simulink model "gm_hdl_model_fixed"  (R2024a)
settings: Solver=FixedStepDiscrete  StartTime=0.0  StopTime=SIM_TIME  RelTol=1e-3
undefined symbols (not defined in the file or in its folder): a, b, BUFFER_LEN, c, SAMPLING_FREQ, signal_1
libraries: hdlsllib x39, dspsigops x15, simulink_extras x4, simulink x2, dspsrcs4 x1, dsphdlxfrm2 x1
(part 3 of 3)

== system gm_hdl_model_fixed/Subsystem1/Subsystem Reference/Real Divide HDL Optimized/ForEach - Real Divide_instance1/Normalize numerator/positiveRealNormalizer/embreciprocals_c3_positiveRealNormalizer_controlled ==
  in0 : Inport  OutDataTypeStr=fixdt(1, 17, 14)  SampleTime=1e-08
  in1 : Inport  Port=2  OutDataTypeStr=boolean  SampleTime=1e-08
  stateControl : EnablePort  OutDataTypeStr=boolean
  embreciprocals_c3_positiveRealNormalizer : MATLAB Function  TreatAsAtomicUnit=on
      settings: LibrarySourceBlock=embreciprocals/Real Normalizer HDL Optimized/positiveRealNormalizer
  out0 : Outport  OutDataTypeStr=fixdt(1, 17, 15)  SampleTime=1e-08  InitialOutput=0
  out1 : Outport  Port=2  OutDataTypeStr=int32  SampleTime=1e-08  InitialOutput=0
  out2 : Outport  Port=3  OutDataTypeStr=boolean  SampleTime=1e-08  InitialOutput=0
  out3 : Outport  Port=4  OutDataTypeStr=boolean  SampleTime=1e-08  InitialOutput=0
  wires:
  embreciprocals_c3_positiveRealNormalizer/1(x) -> out0/1
  embreciprocals_c3_positiveRealNormalizer/2(e) -> out1/1
  embreciprocals_c3_positiveRealNormalizer/3(isNegative) -> out2/1
  embreciprocals_c3_positiveRealNormalizer/4(validOut) -> out3/1
  in0/1 -> embreciprocals_c3_positiveRealNormalizer/1(u)
  in1/1 -> embreciprocals_c3_positiveRealNormalizer/2(validIn)

== matlab function gm_hdl_model_fixed/Subsystem1/Subsystem Reference/Real Divide HDL Optimized/ForEach - Real Divide_instance1/Upcast Wordlength/slutils_c2_Upcast_Wordlength ==
  data: x input; u output; y input; v output
function [u, v] = upcastWordlength(x, y)

% Copyright 2019 The MathWorks, Inc.

%#codegen

[u, v] = fixed.internal.type.upcastWordlength(x,y);

end

== matlab function gm_hdl_model_fixed/Subsystem1/Subsystem Reference/Real Divide HDL Optimized/Reshape to original size/embreciprocals_c11_Reshape_to_original_size ==
  data: y input; u input; z output
function z = reshape_to_original_size(y,u)
    z = reshape(y,size(u));
end

== matlab function gm_hdl_model_fixed/Subsystem1/myRMS/CORDIC Square Root HDL Optimized/Synchronous Subsystem/cordicSquareRootHDL/embmathops_c2_s84XJG1CWMolALoedlonStG_cordicSquareRootHDL_controlled/embmathops_c2_s84XJG1CWMolALoedlonStG_cordicSquareRootHDL ==
  settings: fimath=hdlfimath
  data: u input; dataOut output; validIn input; restart input; eOut output; isZero output; validOut output; maximumShiftValue parameter; nIterPerReg parameter; autoMaximumShiftVal parameter
function [dataOut,eOut,isZero,validOut] = cordicSquareRootHDL(u,validIn,restart,maximumShiftValue, nIterPerReg, autoMaximumShiftVal)
    % [dataOut,eOut,validOut] = cordicSquareRootHDL(u,validIn,restart,maximumShiftValue,nIterPerReg)
    % This function computes the normalized square root of input data u
    % based on CORDIC hyperbolic vectoring mode. eOut is the bit shift
    % value to be used during denormalization.
    %
    % This function first performs normalization of input u and then
    % computes square root of normalized u using CORDIC hyperbolic
    % vectoring mode.

    %   Copyright 2023 The MathWorks, Inc.

    %#codegen
    
    fixed.internal.reciprocal.validateNormalizerInputs(u, validIn);

    %% Constants
    if autoMaximumShiftVal
        N = coder.const(fixed.cordic.maximumShiftValue(u));
    else
        N = coder.const(maximumShiftValue);
    end

    Kn = coder.const(fixed.cordic.hyperbolic.inverseScaleFactor(N));
    INITOFFSET = coder.const(0.25);
    shiftSeq = coder.const(fixed.cordic.hyperbolic.shiftSequence(N));
    nCORDICIterations = coder.const(length(shiftSeq));

    %% Run CORDIC square root workflow
    uPos = fixed.cordic.linear.makeRealScalarPositiveUnsigned(u);
    if isfi(u)&&isscaledtype(u)
        coder.internal.assert(u.WordLength>N,'fixed:emblib:CORDICMaxShiftValMustBeSmallerThanWordlength');
        [dataOut, eOut, isZero, validOut] = sqrtIterFixed(uPos, validIn, restart,nIterPerReg,Kn,INITOFFSET,shiftSeq,nCORDICIterations);
    else
        [dataOut, eOut] = fixed.emblib.cordicsqrt.cordicSqrtFloat(uPos, Kn, INITOFFSET, shiftSeq, nCORDICIterations);
        validOut = validIn;
        isZero = u==0;
    end
end

function [dataOut, eOut, isZero, validOut] = sqrtIterFixed(u, validIn, restart, nIterPerReg, Kn, INITOFFSET, shiftSeq, nCORDICIterations)
        uInt = stripscaling(u);
        
        wordLength = coder.const(uInt.WordLength);
        normalizerType = numerictype(1,32,0);

        % CORDIC datatype and corresponding fimath
        CORDICprototype = fi([],1,wordLength,wordLength-2,'DataType',uInt.DataType);
        Fxy = fixed.fimathLike(CORDICprototype);
        
        % Allocate registers
        [numOfNormSteps,nNormReg,normInd,nTrailingNormSteps,trailingNormIdx,nLeadingCORDICSteps,nCORDICReg,CORDICShiftInd,nTotReg]...
            = fixed.emblib.cordicsqrt.allocateReg(wordLength,nCORDICIterations,nIterPerReg);
        
        %% Registers
        persistent xRegNorm xRegCORDIC yReg eRegNorm eRegCORDIC validReg dataOutReg eOutReg isZeroReg
        if isempty(xRegNorm)
            xRegNorm = zeros(nNormReg,1,'like',uInt);
            xRegCORDIC = setfimath(zeros(nCORDICReg,1,'like',CORDICprototype),Fxy);
            yReg = setfimath(zeros(nCORDICReg,1,'like',CORDICprototype),Fxy);
            eRegNorm = fi(zeros(nNormReg,1),0,numOfNormSteps,0);
            eRegCORDIC = fi(zeros(nCORDICReg,1),normalizerType);
            validReg = false(nTotReg+1,1);
            dataOutReg = setfimath(cast(0,'like',CORDICprototype),Fxy);
            eOutReg = fi(0,normalizerType);
            isZeroReg = false(nTotReg+1,1);
        end
        
        %% Assign outputs
        dataOut = dataOutReg;
        eOut = eOutReg;
        validOut = validReg(end);
        isZero = isZeroReg(end);
        
        %% Update registers
        [xRegNorm, xRegCORDIC, yReg, eRegNorm, eRegCORDIC, validReg, dataOutReg, eOutReg, isZeroReg]...
        = fixed.emblib.cordicsqrt.cordicSqrtFiScaledtypeUpdateReg(u, uInt, validIn, restart,... % Inputs
        xRegNorm, xRegCORDIC, yReg, eRegNorm, eRegCORDIC, validReg, dataOutReg, eOutReg, isZeroReg,... %Registers
        Kn, INITOFFSET, shiftSeq, nIterPerReg,... % Constants for algorithms
        nTotReg, nNormReg, CORDICShiftInd, normInd, nTrailingNormSteps, trailingNormIdx, nLeadingCORDICSteps); % Constants for partition algorithms
end

== matlab function gm_hdl_model_fixed/Subsystem1/Subsystem Reference/Real Divide HDL Optimized/ForEach - Real Divide_instance1/MATLAB Function/embreciprocals_c13_MATLAB_Function ==
  settings: fimath=hdlfimath
  data: num input; num_out output; t_num input; t_num_out output
function [num_out, t_num_out] = fcn(num, t_num)

num_out = bitsra(num,1);
t_num_out = t_num - 1;

end

== matlab function gm_hdl_model_fixed/Subsystem1/myRMS/CORDIC Square Root HDL Optimized/Cast to Union of Types/slutils_c1_sjX4rJHbVvOr6YSpugZXv9B_Cast_to_Union_of_Types ==
  settings: fimath=hdlfimath
  data: Xref input; Cout output; Cin input
function Cout = castToUnionType(Xref,Cin)
    %castToUnionType Cast second input to union of the two types
    if (isfloat(Xref) && isfloat(Cin)) || (isFixed(Xref) && isFixed(Cin))
        T = fixed.internal.type.unionPrototype(Cin,Xref,...
        'RoundingMethod','Floor',...
        'OverflowAction','Wrap');
        Cout = cast(Cin,'like',T);
    else
        coder.internal.assert(false,'fixed:emblib:InputOutputMustBeAllFixedOrFloat');
    end
end

function t = isFixed(x)
    t = (isfi(x) || isa(x,'embedded.numerictype')) && isscalingbinarypoint(x) ...
        || isinteger(x);
end

== matlab function gm_hdl_model_fixed/Subsystem1/myRMS/CORDIC Square Root HDL Optimized/Bit Shift Arithmetic/embmathops_c6_st99WwhDyWfnOmuPiiKPkxE_Bit_Shift_Arithmetic ==
  settings: fimath=hdlfimath
  data: u input; y output; e input; isZero input
function y = bitShiftArithmetic(u,e,isZero)
%#codegen
if isZero
    y = cast(0,'like',u);
else
    if e<0
        y = bitsll(u,-e);
    else
        y = bitsra(u,e);
    end
end

== matlab function gm_hdl_model_fixed/Subsystem1/Subsystem Reference/Absolute of Complex/CORDIC Square Root HDL Optimized1/Cast to Union of Types/slutils_c1_sJq36p6JfwxqYYDPRgb8M6G_Cast_to_Union_of_Types ==
  settings: fimath=hdlfimath
  data: Xref input; Cout output; Cin input
function Cout = castToUnionType(Xref,Cin)
    %castToUnionType Cast second input to union of the two types
    if (isfloat(Xref) && isfloat(Cin)) || (isFixed(Xref) && isFixed(Cin))
        T = fixed.internal.type.unionPrototype(Cin,Xref,...
        'RoundingMethod','Floor',...
        'OverflowAction','Wrap');
        Cout = cast(Cin,'like',T);
    else
        coder.internal.assert(false,'fixed:emblib:InputOutputMustBeAllFixedOrFloat');
    end
end

function t = isFixed(x)
    t = (isfi(x) || isa(x,'embedded.numerictype')) && isscalingbinarypoint(x) ...
        || isinteger(x);
end

== matlab function gm_hdl_model_fixed/Subsystem1/Subsystem Reference/Real Divide HDL Optimized/y = u(1)/embreciprocals_c16_y___u_1_ ==
  data: u input; y output
function y = select_one(u)
    y = u(1);
end

== matlab function gm_hdl_model_fixed/Subsystem1/Subsystem Reference/Real Divide HDL Optimized/Verify divide sizes/embreciprocals_c19_Verify_divide_sizes ==
  data: denominator input; den output; numerator input; num output
function [den,num] = verify_size(denominator,numerator)
   % Verify that the dimensions of the input arrays match, and then reshape
   % them.
   coder.internal.assert(numel(denominator)==numel(numerator),...
       'fixed:emblib:DivideDimensionsShouldMatch',...
       'Real Divide HDL Optimized');
   num = reshape(numerator,1,numel(numerator));
   den = reshape(denominator,1,numel(denominator));
end

== matlab function gm_hdl_model_fixed/Subsystem1/Subsystem Reference/Real Divide HDL Optimized/ForEach - Real Divide_instance1/Divide real numerator by denominator/normalizedCORDICDivide/embreciprocals_c21_normalizedCORDICDivide_controlled/embreciprocals_c21_normalizedCORDICDivide ==
  settings: fimath=hdlfimath
  data: num input; den input; tNum input; tDen input; isNumNegative input; isDenNegative input; y output; t output; isDenZeroOut output; validIn input; validOut output
function [y, t, isDenZeroOut, validOut] = normalizedCORDICDivide(num, den, tNum, tDen, isNumNegative, isDenNegative, validIn)
    %   Copyright 2020 The MathWorks, Inc.
    %#codegen
    fixed.internal.reciprocal.validateReciprocalInputs(num, validIn);
    if isfi(num) && isscaledtype(num)
        isDenZero = den==0;
        isNumZero = num==0;
        % CORDIC divide for fixed-point and scaled-double types
        [y,t,isNegative,isNumZeroOut, isDenZeroOut,validOut] = fixedpointDivide(den,num,tDen-tNum,isNumNegative ~= isDenNegative, isNumZero, isDenZero,validIn);
    else
        % y = num/den for builtin types.
        y = num./den;
        t = tDen - tNum;
        isNegative = isNumNegative ~= isDenNegative;
        validOut = validIn;
        isDenZeroOut = false;
        isNumZeroOut = false;
    end
    if isNumZeroOut
        % Negate with saturate so the most negative value doesn't overflow.
        F = fimath('OverflowAction', 'Saturate');
        y(:) = setfimath(0,F);
    else
        if isNegative
            % Negate with saturate so the most negative value doesn't overflow.
            F = fimath('OverflowAction', 'Saturate');
            y(:) = -setfimath(y,F);
        end
    end
end

function [division, t, isNegativeOut, isNumZeroOut, isDenZeroOut, validOut] = fixedpointDivide(x,y,t_in,isNegative,isNumZero,isDenZero,validIn)
    T = fixed.cordic.linear.positiveReciprocalTypes(x);
    maximumShiftValue = coder.const(fixed.cordic.maximumShiftValue(T.data));
    % Register variables for the CORDIC Divide Kernel
    persistent xReg yReg zReg validReg tReg isNegativeReg isNumZeroReg isDenZeroReg
    if isempty(xReg)
        xReg = zeros(maximumShiftValue+2,1,'like',T.data);
        yReg = zeros(maximumShiftValue+2,1,'like',T.data);
        zReg = zeros(maximumShiftValue+2,1,'like',T.data);
        validReg = zeros(maximumShiftValue+2,1,'like',validIn);
        tReg = zeros(maximumShiftValue+2,1,'like',t_in);
        isNegativeReg = false(maximumShiftValue+2,1);
        isDenZeroReg = false(maximumShiftValue+2,1);
        isNumZeroReg = false(maximumShiftValue+2,1);
    end
    % CORDIC Divide Kernel
    [division,t,validOut,...
        xReg,yReg,zReg,validReg,tReg... % Persistent variables
        ] = fixed.internal.reciprocal.cordicDivideKernel(x,y,t_in,validIn,...
        xReg,yReg,zReg,validReg,tReg... % Persistent variables
        );
    
    % Assign outputs from states
    isNegativeOut = isNegativeReg(end);
    isNumZeroOut = isNumZeroReg(end);
    isDenZeroOut = isDenZeroReg(end);
    % Update isNegative states
    coder.unroll
    for k = maximumShiftValue+1:-1:1
        isNegativeReg(k+1) = isNegativeReg(k);
        isNumZeroReg(k+1) = isNumZeroReg(k);
        isDenZeroReg(k+1) = isDenZeroReg(k);
    end
    isNegativeReg(1) = isNegative;
    isNumZeroReg(1) = isNumZero;
    isDenZeroReg(1) = isDenZero;
end

== matlab function gm_hdl_model_fixed/Subsystem1/Subsystem Reference/Absolute of Complex/CORDIC Square Root HDL Optimized1/Synchronous Subsystem/cordicSquareRootHDL/embmathops_c2_srwrzER3uCGRdPfDbow0ID_cordicSquareRootHDL_controlled/embmathops_c2_srwrzER3uCGRdPfDbow0ID_cordicSquareRootHDL ==
  settings: fimath=hdlfimath
  data: u input; dataOut output; validIn input; restart input; eOut output; isZero output; validOut output; maximumShiftValue parameter; nIterPerReg parameter; autoMaximumShiftVal parameter
function [dataOut,eOut,isZero,validOut] = cordicSquareRootHDL(u,validIn,restart,maximumShiftValue, nIterPerReg, autoMaximumShiftVal)
    % [dataOut,eOut,validOut] = cordicSquareRootHDL(u,validIn,restart,maximumShiftValue,nIterPerReg)
    % This function computes the normalized square root of input data u
    % based on CORDIC hyperbolic vectoring mode. eOut is the bit shift
    % value to be used during denormalization.
    %
    % This function first performs normalization of input u and then
    % computes square root of normalized u using CORDIC hyperbolic
    % vectoring mode.

    %   Copyright 2023 The MathWorks, Inc.

    %#codegen
    
    fixed.internal.reciprocal.validateNormalizerInputs(u, validIn);

    %% Constants
    if autoMaximumShiftVal
        N = coder.const(fixed.cordic.maximumShiftValue(u));
    else
        N = coder.const(maximumShiftValue);
    end

    Kn = coder.const(fixed.cordic.hyperbolic.inverseScaleFactor(N));
    INITOFFSET = coder.const(0.25);
    shiftSeq = coder.const(fixed.cordic.hyperbolic.shiftSequence(N));
    nCORDICIterations = coder.const(length(shiftSeq));

    %% Run CORDIC square root workflow
    uPos = fixed.cordic.linear.makeRealScalarPositiveUnsigned(u);
    if isfi(u)&&isscaledtype(u)
        coder.internal.assert(u.WordLength>N,'fixed:emblib:CORDICMaxShiftValMustBeSmallerThanWordlength');
        [dataOut, eOut, isZero, validOut] = sqrtIterFixed(uPos, validIn, restart,nIterPerReg,Kn,INITOFFSET,shiftSeq,nCORDICIterations);
    else
        [dataOut, eOut] = fixed.emblib.cordicsqrt.cordicSqrtFloat(uPos, Kn, INITOFFSET, shiftSeq, nCORDICIterations);
        validOut = validIn;
        isZero = u==0;
    end
end

function [dataOut, eOut, isZero, validOut] = sqrtIterFixed(u, validIn, restart, nIterPerReg, Kn, INITOFFSET, shiftSeq, nCORDICIterations)
        uInt = stripscaling(u);
        
        wordLength = coder.const(uInt.WordLength);
        normalizerType = numerictype(1,32,0);

        % CORDIC datatype and corresponding fimath
        CORDICprototype = fi([],1,wordLength,wordLength-2,'DataType',uInt.DataType);
        Fxy = fixed.fimathLike(CORDICprototype);
        
        % Allocate registers
        [numOfNormSteps,nNormReg,normInd,nTrailingNormSteps,trailingNormIdx,nLeadingCORDICSteps,nCORDICReg,CORDICShiftInd,nTotReg]...
            = fixed.emblib.cordicsqrt.allocateReg(wordLength,nCORDICIterations,nIterPerReg);
        
        %% Registers
        persistent xRegNorm xRegCORDIC yReg eRegNorm eRegCORDIC validReg dataOutReg eOutReg isZeroReg
        if isempty(xRegNorm)
            xRegNorm = zeros(nNormReg,1,'like',uInt);
            xRegCORDIC = setfimath(zeros(nCORDICReg,1,'like',CORDICprototype),Fxy);
            yReg = setfimath(zeros(nCORDICReg,1,'like',CORDICprototype),Fxy);
            eRegNorm = fi(zeros(nNormReg,1),0,numOfNormSteps,0);
            eRegCORDIC = fi(zeros(nCORDICReg,1),normalizerType);
            validReg = false(nTotReg+1,1);
            dataOutReg = setfimath(cast(0,'like',CORDICprototype),Fxy);
            eOutReg = fi(0,normalizerType);
            isZeroReg = false(nTotReg+1,1);
        end
        
        %% Assign outputs
        dataOut = dataOutReg;
        eOut = eOutReg;
        validOut = validReg(end);
        isZero = isZeroReg(end);
        
        %% Update registers
        [xRegNorm, xRegCORDIC, yReg, eRegNorm, eRegCORDIC, validReg, dataOutReg, eOutReg, isZeroReg]...
        = fixed.emblib.cordicsqrt.cordicSqrtFiScaledtypeUpdateReg(u, uInt, validIn, restart,... % Inputs
        xRegNorm, xRegCORDIC, yReg, eRegNorm, eRegCORDIC, validReg, dataOutReg, eOutReg, isZeroReg,... %Registers
        Kn, INITOFFSET, shiftSeq, nIterPerReg,... % Constants for algorithms
        nTotReg, nNormReg, CORDICShiftInd, normInd, nTrailingNormSteps, trailingNormIdx, nLeadingCORDICSteps); % Constants for partition algorithms
end

== matlab function gm_hdl_model_fixed/Subsystem1/Subsystem Reference/CORDIC Square Root HDL Optimized/Synchronous Subsystem/cordicSquareRootHDL/embmathops_c2_skVmLPFzLIK224pVNfQB1qF_cordicSquareRootHDL_controlled/embmathops_c2_skVmLPFzLIK224pVNfQB1qF_cordicSquareRootHDL ==
  settings: fimath=hdlfimath
  data: u input; dataOut output; validIn input; restart input; eOut output; isZero output; validOut output; maximumShiftValue parameter; nIterPerReg parameter; autoMaximumShiftVal parameter
function [dataOut,eOut,isZero,validOut] = cordicSquareRootHDL(u,validIn,restart,maximumShiftValue, nIterPerReg, autoMaximumShiftVal)
    % [dataOut,eOut,validOut] = cordicSquareRootHDL(u,validIn,restart,maximumShiftValue,nIterPerReg)
    % This function computes the normalized square root of input data u
    % based on CORDIC hyperbolic vectoring mode. eOut is the bit shift
    % value to be used during denormalization.
    %
    % This function first performs normalization of input u and then
    % computes square root of normalized u using CORDIC hyperbolic
    % vectoring mode.

    %   Copyright 2023 The MathWorks, Inc.

    %#codegen
    
    fixed.internal.reciprocal.validateNormalizerInputs(u, validIn);

    %% Constants
    if autoMaximumShiftVal
        N = coder.const(fixed.cordic.maximumShiftValue(u));
    else
        N = coder.const(maximumShiftValue);
    end

    Kn = coder.const(fixed.cordic.hyperbolic.inverseScaleFactor(N));
    INITOFFSET = coder.const(0.25);
    shiftSeq = coder.const(fixed.cordic.hyperbolic.shiftSequence(N));
    nCORDICIterations = coder.const(length(shiftSeq));

    %% Run CORDIC square root workflow
    uPos = fixed.cordic.linear.makeRealScalarPositiveUnsigned(u);
    if isfi(u)&&isscaledtype(u)
        coder.internal.assert(u.WordLength>N,'fixed:emblib:CORDICMaxShiftValMustBeSmallerThanWordlength');
        [dataOut, eOut, isZero, validOut] = sqrtIterFixed(uPos, validIn, restart,nIterPerReg,Kn,INITOFFSET,shiftSeq,nCORDICIterations);
    else
        [dataOut, eOut] = fixed.emblib.cordicsqrt.cordicSqrtFloat(uPos, Kn, INITOFFSET, shiftSeq, nCORDICIterations);
        validOut = validIn;
        isZero = u==0;
    end
end

function [dataOut, eOut, isZero, validOut] = sqrtIterFixed(u, validIn, restart, nIterPerReg, Kn, INITOFFSET, shiftSeq, nCORDICIterations)
        uInt = stripscaling(u);
        
        wordLength = coder.const(uInt.WordLength);
        normalizerType = numerictype(1,32,0);

        % CORDIC datatype and corresponding fimath
        CORDICprototype = fi([],1,wordLength,wordLength-2,'DataType',uInt.DataType);
        Fxy = fixed.fimathLike(CORDICprototype);
        
        % Allocate registers
        [numOfNormSteps,nNormReg,normInd,nTrailingNormSteps,trailingNormIdx,nLeadingCORDICSteps,nCORDICReg,CORDICShiftInd,nTotReg]...
            = fixed.emblib.cordicsqrt.allocateReg(wordLength,nCORDICIterations,nIterPerReg);
        
        %% Registers
        persistent xRegNorm xRegCORDIC yReg eRegNorm eRegCORDIC validReg dataOutReg eOutReg isZeroReg
        if isempty(xRegNorm)
            xRegNorm = zeros(nNormReg,1,'like',uInt);
            xRegCORDIC = setfimath(zeros(nCORDICReg,1,'like',CORDICprototype),Fxy);
            yReg = setfimath(zeros(nCORDICReg,1,'like',CORDICprototype),Fxy);
            eRegNorm = fi(zeros(nNormReg,1),0,numOfNormSteps,0);
            eRegCORDIC = fi(zeros(nCORDICReg,1),normalizerType);
            validReg = false(nTotReg+1,1);
            dataOutReg = setfimath(cast(0,'like',CORDICprototype),Fxy);
            eOutReg = fi(0,normalizerType);
            isZeroReg = false(nTotReg+1,1);
        end
        
        %% Assign outputs
        dataOut = dataOutReg;
        eOut = eOutReg;
        validOut = validReg(end);
        isZero = isZeroReg(end);
        
        %% Update registers
        [xRegNorm, xRegCORDIC, yReg, eRegNorm, eRegCORDIC, validReg, dataOutReg, eOutReg, isZeroReg]...
        = fixed.emblib.cordicsqrt.cordicSqrtFiScaledtypeUpdateReg(u, uInt, validIn, restart,... % Inputs
        xRegNorm, xRegCORDIC, yReg, eRegNorm, eRegCORDIC, validReg, dataOutReg, eOutReg, isZeroReg,... %Registers
        Kn, INITOFFSET, shiftSeq, nIterPerReg,... % Constants for algorithms
        nTotReg, nNormReg, CORDICShiftInd, normInd, nTrailingNormSteps, trailingNormIdx, nLeadingCORDICSteps); % Constants for partition algorithms
end

== matlab function gm_hdl_model_fixed/Subsystem1/Subsystem Reference/CORDIC Square Root HDL Optimized/Cast to Union of Types/slutils_c1_sUkuwzpcxqKl25e4GzDa0OH_Cast_to_Union_of_Types ==
  settings: fimath=hdlfimath
  data: Xref input; Cout output; Cin input
function Cout = castToUnionType(Xref,Cin)
    %castToUnionType Cast second input to union of the two types
    if (isfloat(Xref) && isfloat(Cin)) || (isFixed(Xref) && isFixed(Cin))
        T = fixed.internal.type.unionPrototype(Cin,Xref,...
        'RoundingMethod','Floor',...
        'OverflowAction','Wrap');
        Cout = cast(Cin,'like',T);
    else
        coder.internal.assert(false,'fixed:emblib:InputOutputMustBeAllFixedOrFloat');
    end
end

function t = isFixed(x)
    t = (isfi(x) || isa(x,'embedded.numerictype')) && isscalingbinarypoint(x) ...
        || isinteger(x);
end

== matlab function gm_hdl_model_fixed/Subsystem1/Subsystem Reference/CORDIC Square Root HDL Optimized/Bit Shift Arithmetic/embmathops_c6_sxviEMGenxpVSWTChSq0GHG_Bit_Shift_Arithmetic ==
  settings: fimath=hdlfimath
  data: u input; y output; e input; isZero input
function y = bitShiftArithmetic(u,e,isZero)
%#codegen
if isZero
    y = cast(0,'like',u);
else
    if e<0
        y = bitsll(u,-e);
    else
        y = bitsra(u,e);
    end
end

== matlab function gm_hdl_model_fixed/Subsystem1/Subsystem Reference/Absolute of Complex/CORDIC Square Root HDL Optimized1/Bit Shift Arithmetic/embmathops_c6_s5qJlWhB5AyunXvC1Wsa7cH_Bit_Shift_Arithmetic ==
  settings: fimath=hdlfimath
  data: u input; y output; e input; isZero input
function y = bitShiftArithmetic(u,e,isZero)
%#codegen
if isZero
    y = cast(0,'like',u);
else
    if e<0
        y = bitsll(u,-e);
    else
        y = bitsra(u,e);
    end
end

== matlab function gm_hdl_model_fixed/Subsystem1/Subsystem Reference/Real Divide HDL Optimized/ForEach - Real Divide_instance1/Shift and cast to output type/Cast to Union of Types/slutils_c1_sfkclysknIFh6pVVpTDebQG_Cast_to_Union_of_Types ==
  settings: fimath=hdlfimath
  data: Xref input; Cout output; Cin input
function Cout = castToUnionType(Xref,Cin)
    %castToUnionType Cast second input to union of the two types
    if (isfloat(Xref) && isfloat(Cin)) || (isFixed(Xref) && isFixed(Cin))
        T = fixed.internal.type.unionPrototype(Cin,Xref,...
        'RoundingMethod','Floor',...
        'OverflowAction','Wrap');
        Cout = cast(Cin,'like',T);
    else
        coder.internal.assert(false,'fixed:emblib:InputOutputMustBeAllFixedOrFloat');
    end
end

function t = isFixed(x)
    t = (isfi(x) || isa(x,'embedded.numerictype')) && isscalingbinarypoint(x) ...
        || isinteger(x);
end

== matlab function gm_hdl_model_fixed/Subsystem1/Subsystem Reference/Real Divide HDL Optimized/ForEach - Real Divide_instance1/Normalize numerator/positiveRealNormalizer/embreciprocals_c3_positiveRealNormalizer_controlled/embreciprocals_c3_positiveRealNormalizer ==
  settings: fimath=hdlfimath
  data: u input; x output; validIn input; e output; isNegative output; validOut output
function [x, e, isNegative, validOut] = realNormalizer(u, validIn)
    %realNormalizer Normalize real values.
    % Given real scalar u ~= 0, this block produces x such that
    %    1 <= x < 2,
    % e such that
    %    x = (2^e)*|u|,
    % and isNegative = u<0.
    %
    %   When u = 0 and u is fixed-point or scaled-double, then x = 0 and
    %   e = (2^nextpow2(x.WordLength)) - x.WordLength - x.FractionLength.
    %
    %   When u = 0 and u is floating-point, then x = 0 and e = 1.
    
    %   Copyright 2019 The MathWorks, Inc.
    %#codegen
    
    % This function only works on scalars.
    % Only operate on the real part
    fixed.internal.reciprocal.validateNormalizerInputs(u, validIn);
    % Normalize in unsigned type.
    [x_normalized, n_normalized, isNegative, validOut] = normalize(real(u), validIn);
    % Cast the output to signed if the input was signed.
    x = fixed.internal.reciprocal.castToInputSignedness(x_normalized,u);
    % Convert the normalized shift value based on the data type of the
    % input U so that the output of the normalizer X is in real-world
    % scale and X = (2^N)*U.
    e = fi(int32(0));
    e(:) = fixed.internal.reciprocal.normalizedShiftToRealWorldValueShift(n_normalized,u);
end

function [x_normalized, e_normalized, isNegative, validOut] = normalize(u, validIn)
    [u, isNegative] = fixed.reciprocal.pipelined.makeRealScalarPositive(u);
    if isfi(u) && isfixed(u)
        % Normalize fixed-point values
        [x_normalized, e_normalized, isNegative, validOut] = normalizeFixedpoint(u, isNegative, validIn);
    else
        % Normalize floating-point or scaled-double
        [x_normalized, e_normalized, validOut] = fixed.internal.reciprocal.normalizePositiveFloatOrScaledDouble(u, validIn);
    end
end

function [u_normalized, e_normalized, isNegativeOut, validOut] = normalizeFixedpoint(u, isNegative, validIn)
    % Normalize fixed-point values.
    persistent validReg
    persistent tReg
    persistent xReg
    persistent isNegativeReg
    % For fixed-point types, the normalization uses a binary search of
    % length log2 of the word length of the input.
    number_of_stages = coder.const(nextpow2(u.WordLength));
    
    if isempty(validReg)
        validReg = false(number_of_stages+1,1);
        tReg = zeros(number_of_stages+1,1,'like',fi(0,0,max(number_of_stages,1),0));
        xReg = zeros(number_of_stages+1,1,'like',fi([],0,u.WordLength,0));
        isNegativeReg = false(number_of_stages+1,1);
    end
    
    [u_normalized, e_normalized,validOut,...
        validReg, tReg,xReg...  % Persistent
        ] = fixed.internal.reciprocal.normalizePositiveFixedPoint(u, validIn, number_of_stages, ...
        validReg, tReg,xReg...  % Persistent
        );
    % Assign outputs from states
    isNegativeOut = isNegativeReg(end);
    
    % Update isNegative states
    coder.unroll;
    for k = number_of_stages:-1:1
        isNegativeReg(k+1) = isNegativeReg(k);
    end
    isNegativeReg(1) = isNegative;
end

== matlab function gm_hdl_model_fixed/Subsystem1/Subsystem Reference/Real Divide HDL Optimized/ForEach - Real Divide_instance1/Normalize denominator/positiveRealNormalizer/embreciprocals_c3_positiveRealNormalizer_controlled/embreciprocals_c3_positiveRealNormalizer ==
  settings: fimath=hdlfimath
  data: u input; x output; validIn input; e output; isNegative output; validOut output
function [x, e, isNegative, validOut] = realNormalizer(u, validIn)
    %realNormalizer Normalize real values.
    % Given real scalar u ~= 0, this block produces x such that
    %    1 <= x < 2,
    % e such that
    %    x = (2^e)*|u|,
    % and isNegative = u<0.
    %
    %   When u = 0 and u is fixed-point or scaled-double, then x = 0 and
    %   e = (2^nextpow2(x.WordLength)) - x.WordLength - x.FractionLength.
    %
    %   When u = 0 and u is floating-point, then x = 0 and e = 1.
    
    %   Copyright 2019 The MathWorks, Inc.
    %#codegen
    
    % This function only works on scalars.
    % Only operate on the real part
    fixed.internal.reciprocal.validateNormalizerInputs(u, validIn);
    % Normalize in unsigned type.
    [x_normalized, n_normalized, isNegative, validOut] = normalize(real(u), validIn);
    % Cast the output to signed if the input was signed.
    x = fixed.internal.reciprocal.castToInputSignedness(x_normalized,u);
    % Convert the normalized shift value based on the data type of the
    % input U so that the output of the normalizer X is in real-world
    % scale and X = (2^N)*U.
    e = fi(int32(0));
    e(:) = fixed.internal.reciprocal.normalizedShiftToRealWorldValueShift(n_normalized,u);
end

function [x_normalized, e_normalized, isNegative, validOut] = normalize(u, validIn)
    [u, isNegative] = fixed.reciprocal.pipelined.makeRealScalarPositive(u);
    if isfi(u) && isfixed(u)
        % Normalize fixed-point values
        [x_normalized, e_normalized, isNegative, validOut] = normalizeFixedpoint(u, isNegative, validIn);
    else
        % Normalize floating-point or scaled-double
        [x_normalized, e_normalized, validOut] = fixed.internal.reciprocal.normalizePositiveFloatOrScaledDouble(u, validIn);
    end
end

function [u_normalized, e_normalized, isNegativeOut, validOut] = normalizeFixedpoint(u, isNegative, validIn)
    % Normalize fixed-point values.
    persistent validReg
    persistent tReg
    persistent xReg
    persistent isNegativeReg
    % For fixed-point types, the normalization uses a binary search of
    % length log2 of the word length of the input.
    number_of_stages = coder.const(nextpow2(u.WordLength));
    
    if isempty(validReg)
        validReg = false(number_of_stages+1,1);
        tReg = zeros(number_of_stages+1,1,'like',fi(0,0,max(number_of_stages,1),0));
        xReg = zeros(number_of_stages+1,1,'like',fi([],0,u.WordLength,0));
        isNegativeReg = false(number_of_stages+1,1);
    end
    
    [u_normalized, e_normalized,validOut,...
        validReg, tReg,xReg...  % Persistent
        ] = fixed.internal.reciprocal.normalizePositiveFixedPoint(u, validIn, number_of_stages, ...
        validReg, tReg,xReg...  % Persistent
        );
    % Assign outputs from states
    isNegativeOut = isNegativeReg(end);
    
    % Update isNegative states
    coder.unroll;
    for k = number_of_stages:-1:1
        isNegativeReg(k+1) = isNegativeReg(k);
    end
    isNegativeReg(1) = isNegative;
end
